simulink subsystem "Actuator_RW"  (R2025a)
settings: Solver=VariableStepAuto  StartTime=0.0  StopTime=10.0  RelTol=1e-3
undefined symbols (not defined in the file): config
settings Model: Creator=Jackt  LastModifiedBy=Jackt

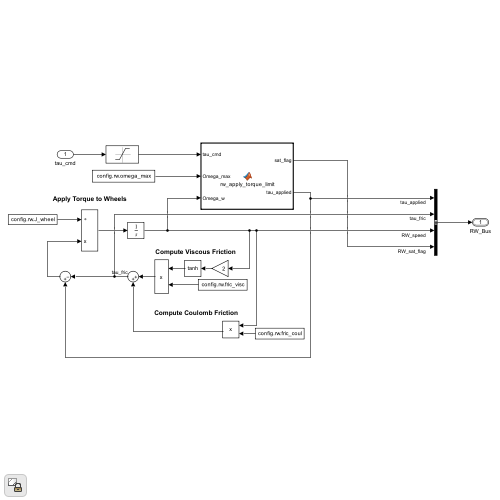
[thumbnail: Simulink's stored preview of the top-level diagram]
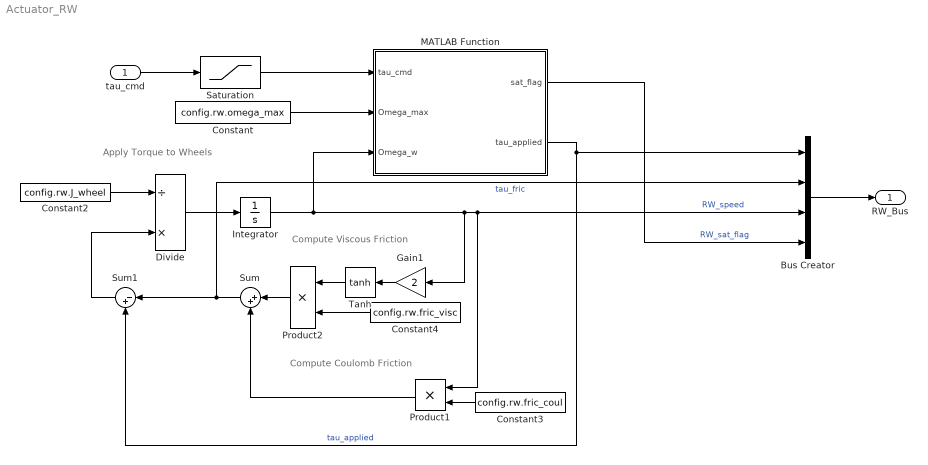
== system Actuator_RW ==
  note: Apply Torque to Wheels
  note: Compute Viscous Friction
  note: Compute Coulomb Friction
  tau_cmd : Inport
  Bus Creator : BusCreator  Inputs=4  OutDataTypeStr=Bus: reactionWheelBus
  Constant : Constant  Value=config.rw.omega_max  VectorParams1D=off
  Constant2 : Constant  Value=config.rw.J_wheel  VectorParams1D=off
  Constant3 : Constant  Value=config.rw.fric_coul  VectorParams1D=off
  Constant4 : Constant  Value=config.rw.fric_visc  VectorParams1D=off
  Divide : Product  Inputs=/*
  Gain1 : Gain  Gain=2
  Integrator : Integrator
  MATLAB Function : MATLAB Function  TreatAsAtomicUnit=on
  Product1 : Product
  Product2 : Product
  Saturation : Saturate  UpperLimit=config.rw.tau_max  LowerLimit=-config.rw.tau_max
  Sum : Sum  Inputs=|++
  Sum1 : Sum  Inputs=|-+
  Tanh : Trigonometry  Operator=tanh
  RW_Bus : Outport  OutDataTypeStr=Bus: reactionWheelBus
  wires:
  Saturation/1 -> MATLAB Function/1(tau_cmd)
  tau_cmd/1 -> Saturation/1
  Integrator/1 -> MATLAB Function/3(Omega_w), Product1/1, Bus Creator/3, Gain1/1  "RW_speed"
  Divide/1 -> Integrator/1
  MATLAB Function/1(sat_flag) -> Bus Creator/4  "RW_sat_flag"
  Constant/1 -> MATLAB Function/2(Omega_max)
  Constant3/1 -> Product1/2
  Gain1/1 -> Tanh/1
  Tanh/1 -> Product2/1
  Constant4/1 -> Product2/2
  Product2/1 -> Sum/1
  Product1/1 -> Sum/2
  Sum/1 -> Sum1/1, Bus Creator/2  "tau_fric"
  MATLAB Function/2(tau_applied) -> Bus Creator/1, Sum1/2  "tau_applied"
  Sum1/1 -> Divide/2
  Constant2/1 -> Divide/1
  Bus Creator/1 -> RW_Bus/1

== matlab function Actuator_RW/MATLAB Function ==
  data: sat_flag output; tau_cmd input; tau_applied output; Omega_max input; Omega_w input
function [sat_flag, tau_applied]   = rw_apply_torque_limit(tau_cmd, Omega_max, Omega_w)
%RW_APPLY_TORQUE_LIMIT

%Force shapes
tau_cmd  = reshape(tau_cmd,  [3 1]);
Omega_w  = reshape(Omega_w,  [3 1]);

%Preallocate output
tau_applied = zeros(3,1);
sat_flag = zeros(3, 1);

%Small tolerance to avoid chattering at the limit
tol = 1e-6;

%Axis-by-axis limiting
for i = 1:3
    tau_i = tau_cmd(i);
    omega_i = Omega_w(i);

    %If wheel is at/over +Omega_max AND commanded torque would increase speed -> block
    if (omega_i >= (Omega_max - tol) && tau_i > 0)
        tau_applied(i) = 0;
        sat_flag(i) = 1;

    %If wheel is at/over -Omega_max AND commanded torque would decrease speed further -> block
    elseif (omega_i <= (-Omega_max + tol) && tau_i < 0)
        tau_applied(i) = 0;
        sat_flag(i) = 1;

    %Otherwise allow commanded torque
    else
        tau_applied(i) = tau_i;
    end
end

end
